simulink model "DCMotorSpeedControl3"  (Simulink 8.9)
settings: Solver=ode45  StartTime=0.0  StopTime=10  RelTol=1e-3  EnableMultiTasking=on
undefined symbols (not defined in the file): B, J, Ke, Kt, La, Ra
settings Model: Creator=page365  LastModifiedBy=edward
settings OptimizationCC: ExpressionDepthLimit=2147483647
settings DebuggingCC: SolverPrmCheckMsg=warning

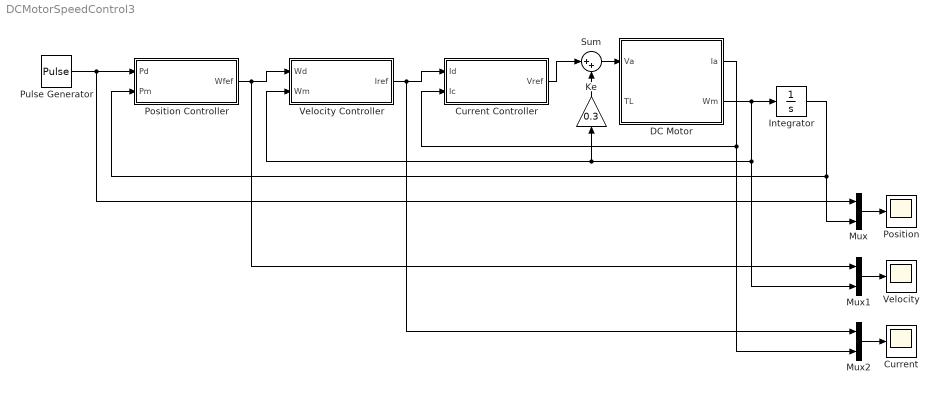
== system DCMotorSpeedControl3 ==
  Current : Scope
  Current Controller : Subsystem
  DC Motor : Subsystem
  Integrator : Integrator
  Ke : Gain  Gain=0.3
  Mux : Mux  Inputs=2
  Mux1 : Mux  Inputs=2
  Mux2 : Mux  Inputs=2
  Position : Scope
  Position Controller : Subsystem
  Pulse Generator : DiscretePulseGenerator  PulseType=Time based  Amplitude=100  Period=10  PulseWidth=50  PhaseDelay=1
  Sum : Sum  Inputs=|++
  Velocity : Scope
  Velocity Controller : Subsystem
  wires:
  Mux/1 -> Position/1
  DC Motor/1(Ia) -> Current Controller/2(Ic), Mux2/2
  Velocity Controller/1(Iref) -> Current Controller/1(Id), Mux2/1
  DC Motor/2(Wm) -> Integrator/1, Mux1/2, Velocity Controller/2(Wm), Ke/1
  Integrator/1 -> Position Controller/2(Pm), Mux/2
  Position Controller/1(Wfef) -> Velocity Controller/1(Wd), Mux1/1
  Pulse Generator/1 -> Position Controller/1(Pd), Mux/1
  Mux1/1 -> Velocity/1
  Mux2/1 -> Current/1
  Current Controller/1(Vref) -> Sum/1
  Sum/1 -> DC Motor/1(Va)
  Ke/1 -> Sum/2

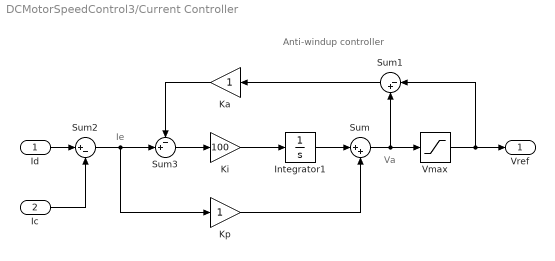
== system DCMotorSpeedControl3/Current Controller ==
  note: Anti-windup controller
  note: Ie
  note: Va
  Id : Inport
  Ic : Inport  Port=2
  Integrator1 : Integrator
  Ka : Gain
  Ki : Gain  Gain=100
  Kp : Gain
  Sum : Sum  Inputs=|++
  Sum1 : Sum  Inputs=|-+
  Sum2 : Sum  Inputs=|+-
  Sum3 : Sum  Inputs=-+|
  Vmax : Saturate  UpperLimit=20  LowerLimit=-20
  Vref : Outport
  wires:
  Vmax/1 -> Sum1/1, Vref/1
  Kp/1 -> Sum/2
  Integrator1/1 -> Sum/1
  Ki/1 -> Integrator1/1
  Sum/1 -> Vmax/1, Sum1/2
  Sum1/1 -> Ka/1
  Ka/1 -> Sum3/1
  Sum3/1 -> Ki/1
  Sum2/1 -> Sum3/2, Kp/1
  Id/1 -> Sum2/1
  Ic/1 -> Sum2/2

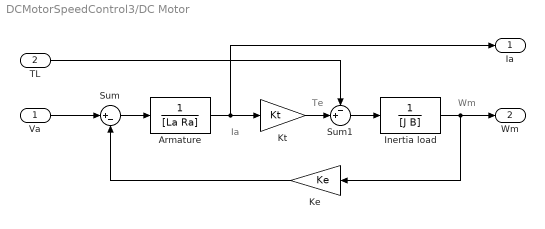
== system DCMotorSpeedControl3/DC Motor ==
  note: Ia
  note: Te
  note: Wm
  Va : Inport
  TL : Inport  Port=2
  Armature : TransferFcn  Denominator=[La Ra]
  Inertia load : TransferFcn  Denominator=[J B]
  Ke : Gain  Gain=Ke
  Kt : Gain  Gain=Kt
  Sum : Sum  Inputs=|+-
  Sum1 : Sum  Inputs=-+|
  Ia : Outport
  Wm : Outport  Port=2
  wires:
  Inertia load/1 -> Ke/1, Wm/1
  Sum1/1 -> Inertia load/1
  Armature/1 -> Kt/1, Ia/1
  Sum/1 -> Armature/1
  Ke/1 -> Sum/2
  Va/1 -> Sum/1
  TL/1 -> Sum1/1
  Kt/1 -> Sum1/2

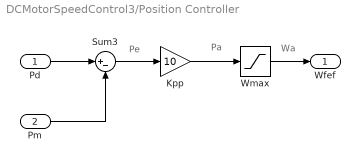
== system DCMotorSpeedControl3/Position Controller ==
  note: Pe
  note: Pa
  note: Wa
  Pd : Inport
  Pm : Inport  Port=2
  Kpp : Gain  Gain=10
  Sum3 : Sum  Inputs=|+-
  Wmax : Saturate  UpperLimit=100  LowerLimit=-100
  Wfef : Outport
  wires:
  Kpp/1 -> Wmax/1
  Pd/1 -> Sum3/1
  Sum3/1 -> Kpp/1
  Pm/1 -> Sum3/2
  Wmax/1 -> Wfef/1

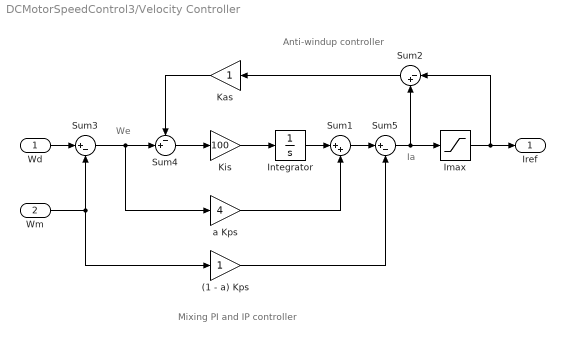
== system DCMotorSpeedControl3/Velocity Controller ==
  note: Mixing PI and IP controller
  note: Anti-windup controller
  note: Ia
  note: We
  Wd : Inport
  Wm : Inport  Port=2
  (1 - a) Kps : Gain
  Imax : Saturate  UpperLimit=20  LowerLimit=-20
  Integrator : Integrator
  Kas : Gain
  Kis : Gain  Gain=100
  Sum1 : Sum  Inputs=|++
  Sum2 : Sum  Inputs=|-+
  Sum3 : Sum  Inputs=|+-
  Sum4 : Sum  Inputs=-+|
  Sum5 : Sum  Inputs=|+-
  a Kps : Gain  Gain=4
  Iref : Outport
  wires:
  Kis/1 -> Integrator/1
  Sum3/1 -> a Kps/1, Sum4/2
  Wd/1 -> Sum3/1
  Wm/1 -> Sum3/2, (1 - a) Kps/1
  Sum5/1 -> Imax/1, Sum2/2
  Imax/1 -> Iref/1, Sum2/1
  Sum2/1 -> Kas/1
  Kas/1 -> Sum4/1
  Sum4/1 -> Kis/1
  Sum1/1 -> Sum5/1
  Integrator/1 -> Sum1/1
  a Kps/1 -> Sum1/2
  (1 - a) Kps/1 -> Sum5/2
